simulink model "evolution_T_acausal"  (R2021a)
settings: Solver=VariableStepAuto  StartTime=0.0  StopTime=2000000  RelTol=1e-3
undefined symbols (not defined in the file): e_mur, ro_baie, ro_mur, S_haut, S_laterale, S_mur, Text, v_baie, v_mur
libraries: fl_lib x15, nesl_utility x2
settings Model: Creator=ethan  LastModifiedBy=ethan
settings SolverCC: AlgebraicLoopSolver=TrustRegion

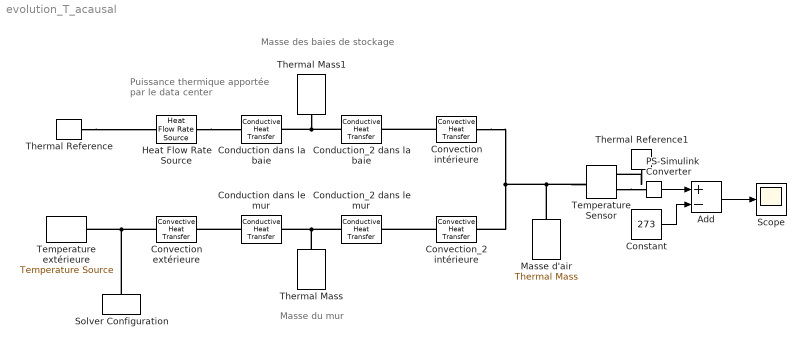
== system evolution_T_acausal ==
  note: Masse du mur
  note: Masse des baies de stockage
  note: Puissance thermique
      | apportée par le data
      | 	     center
  " Masse d'air" : fl_lib/Thermal/Thermal Elements/Thermal Mass  mass=1000*25 kg  sp_heat=1012 J/kg/K  T_specify=on  T_priority=High  T=Text K  T_nominal_specify=off  T_nominal_unit=K  T_nominal_value=1  Q_specify=off  Q_priority=None  Q=0 W  Q_nominal_specify=off  Q_nominal_unit=W  Q_nominal_value=1
  Add : Sum  Inputs=+-
  Conduction dans la baie : fl_lib/Thermal/Thermal Elements/Conductive Heat Transfer  area=4*S_laterale+S_haut m^2  thickness=e_baie m  th_cond=lambda_baie W/(m*K)  T_specify=off  T_priority=None  T=0 K  T_nominal_specify=off  T_nominal_unit=K  T_nominal_value=1  Q_specify=off  Q_priority=None  Q=0 W  Q_nominal_specify=off  Q_nominal_unit=W  Q_nominal_value=1
  Conduction dans le mur : fl_lib/Thermal/Thermal Elements/Conductive Heat Transfer  area=4*S_mur m^2  thickness=e_mur/2 m  th_cond=lambda_mur W/(m*K)  T_specify=off  T_priority=None  T=0 K  T_nominal_specify=off  T_nominal_unit=K  T_nominal_value=1  Q_specify=off  Q_priority=None  Q=0 W  Q_nominal_specify=off  Q_nominal_unit=W  Q_nominal_value=1
  Conduction_2 dans la baie : fl_lib/Thermal/Thermal Elements/Conductive Heat Transfer  area=4*S_laterale+S_haut m^2  thickness=e_baie m  th_cond=lambda_baie W/(m*K)  T_specify=off  T_priority=None  T=0 K  T_nominal_specify=off  T_nominal_unit=K  T_nominal_value=1  Q_specify=off  Q_priority=None  Q=0 W  Q_nominal_specify=off  Q_nominal_unit=W  Q_nominal_value=1
  Conduction_2 dans le mur : fl_lib/Thermal/Thermal Elements/Conductive Heat Transfer  area=4*S_mur m^2  thickness=e_mur/2 m  th_cond=lambda_mur W/(m*K)  T_specify=off  T_priority=None  T=0 K  T_nominal_specify=off  T_nominal_unit=K  T_nominal_value=1  Q_specify=off  Q_priority=None  Q=0 W  Q_nominal_specify=off  Q_nominal_unit=W  Q_nominal_value=1
  Constant : Constant  Value=273
  Convection extérieure : fl_lib/Thermal/Thermal Elements/Convective Heat Transfer  area=4*S_mur m^2  heat_tr_coeff=h_air W/(m^2 * K)  T_specify=off  T_priority=None  T=0 K  T_nominal_specify=off  T_nominal_unit=K  T_nominal_value=1  Q_specify=off  Q_priority=None  Q=0 W  Q_nominal_specify=off  Q_nominal_unit=W  Q_nominal_value=1
      settings: LogSimulationData=on
  Convection intérieure : fl_lib/Thermal/Thermal Elements/Convective Heat Transfer  area=4*S_laterale+S_haut m^2  heat_tr_coeff=h_air W/(m^2 * K)  T_specify=off  T_priority=None  T=0 K  T_nominal_specify=off  T_nominal_unit=K  T_nominal_value=1  Q_specify=off  Q_priority=None  Q=0 W  Q_nominal_specify=off  Q_nominal_unit=W  Q_nominal_value=1
      settings: LogSimulationData=on
  Convection_2 intérieure : fl_lib/Thermal/Thermal Elements/Convective Heat Transfer  area=4*S_mur m^2  heat_tr_coeff=h_air W/(m^2 * K)  T_specify=off  T_priority=None  T=0 K  T_nominal_specify=off  T_nominal_unit=K  T_nominal_value=1  Q_specify=off  Q_priority=None  Q=0 W  Q_nominal_specify=off  Q_nominal_unit=W  Q_nominal_value=1
      settings: LogSimulationData=on
  Heat Flow Rate Source : fl_lib/Thermal/Thermal Sources/Heat Flow Rate Source  heat_flow=P_data W
      settings: SourceProductBaseCode=SS  InternalSimscapePortConfiguration="{\"Bottom\":[],\"Left\":[{\"id\":\"B\",\"label\":\"B\",\"type\":\"foundation.thermal.thermal\"}],\"Right\":[{\"id\":\"A\",\"label\":\"A\",\"type\":\"foundation.thermal.thermal\"}],\"Top\":[]}"
  PS-Simulink Converter : nesl_utility/PS-Simulink Converter  PhysicalDomain=network_engine_domain  SubClassName=ps_output  LeftPortType=input  RightPortType=output  PseudoPeriodic=off  Frequencies=[]  Unit=inherit  AffineConversion=off
      settings: SourceProductBaseCode=PW,SS
  Scope : Scope
  Solver Configuration : nesl_utility/Solver Configuration  PhysicalDomain=network_engine_domain  SubClassName=solver  LeftPortType=input  RightPortType=generic  Tones=[]  Harmonics=[]  SimulateNoise=off  Profile=off  UseLocalSampling=off  EnableSwitchedLinearOptims=on  FrequencyDomain=off  UseCCode=off  RelTol=0.001  AbsTol=1e-06  MinStep=1e-09  ToWorkspace=off  RevertToSquareIcSolve=off  NumHomotopyIterations=100  PhasorMode=off  PhasorModeNumHarmonics=1  DoDC=off  ResidualTolerance=1e-09  UseLocalSolver=off  LocalSolverChoice=NE_BACKWARD_EULER_ADVANCER  LocalSolverSampleTime=0.001  DoFixedCost=off  MaxNonlinIter=3  MaxModeIter=2  ComputeImpulses=off  ImpulseIterations=2  LinearAlgebra=auto  EquationFormulation=NE_TIME_EF  DelaysMemoryBudget=1024  AutomaticFiltering=on  FilteringTimeConstant=0.001  PartitionStorageMethod=AS_NEEDED  PartitionMemoryBudget=1024  PartitionMethod=ROBUST
      settings: SourceProductBaseCode=PW,SS
  Temperature extérieure : fl_lib/Thermal/Thermal Sources/Temperature Source  temperature=Text K
  Temperature Sensor : fl_lib/Thermal/Thermal Sensors/Temperature Sensor
  Thermal Mass : fl_lib/Thermal/Thermal Elements/Thermal Mass  mass=ro_mur*v_mur kg  sp_heat=Cp_mur J/kg/K  T_specify=on  T_priority=High  T=Text K  T_nominal_specify=off  T_nominal_unit=K  T_nominal_value=1  Q_specify=off  Q_priority=None  Q=0 W  Q_nominal_specify=off  Q_nominal_unit=W  Q_nominal_value=1
  Thermal Mass1 : fl_lib/Thermal/Thermal Elements/Thermal Mass  mass=ro_baie*v_baie kg  sp_heat=Cp_baie J/kg/K  T_specify=on  T_priority=High  T=Text K  T_nominal_specify=off  T_nominal_unit=K  T_nominal_value=1  Q_specify=off  Q_priority=None  Q=0 W  Q_nominal_specify=off  Q_nominal_unit=W  Q_nominal_value=1
  Thermal Reference : fl_lib/Thermal/Thermal Elements/Thermal Reference
  Thermal Reference1 : fl_lib/Thermal/Thermal Elements/Thermal Reference
  wires:
  PS-Simulink Converter/1 -> Add/1
  Add/1 -> Scope/1
  Constant/1 -> Add/2
  connections:
  Thermal Mass/LConn1 -- Conduction_2 dans le mur/LConn1 -- Conduction dans le mur/RConn1
  Temperature Sensor/LConn1 -- " Masse d'air"/LConn1 -- Convection intérieure/RConn1 -- Convection_2 intérieure/RConn1
  Convection_2 intérieure/LConn1 -- Conduction_2 dans le mur/RConn1
  Conduction dans le mur/LConn1 -- Convection extérieure/RConn1
  Convection extérieure/LConn1 -- Solver Configuration/RConn1 -- Temperature extérieure/LConn1
  Temperature Sensor/RConn2 -- PS-Simulink Converter/LConn1
  Thermal Reference1/LConn1 -- Temperature Sensor/RConn1
  Thermal Reference/LConn1 -- Heat Flow Rate Source/RConn1
  Conduction_2 dans la baie/LConn1 -- Thermal Mass1/LConn1 -- Conduction dans la baie/RConn1
  Heat Flow Rate Source/LConn1 -- Conduction dans la baie/LConn1
  Convection intérieure/LConn1 -- Conduction_2 dans la baie/RConn1
